simulink model "overhead_crane_control"  (R2022a)
settings: Solver=ode45  StartTime=0.0  StopTime=50  FixedStep=0.001  MaxStep=0.1  MinStep=0.01  RelTol=1e-3  AbsTol=0.01  EnableMultiTasking=on
undefined symbols (not defined in the file): g, k, Kde, Ke, Ku, l, ml, mt, sigbuilder_block
libraries: fuzblock x1
settings Model: Creator=Сергей  LastModifiedBy=clever0ne
settings SolverCC: InitialStep=0.01  ZeroCrossAlgorithm=Adaptive  AlgebraicLoopSolver=TrustRegion
settings DataIOCC: SaveFormat=Array  ReturnWorkspaceOutputs=off
settings OptimizationCC: LifeSpan=inf
settings DebuggingCC: IgnoredZcDiagnostic=none  UnconnectedInputMsg=warning  UnconnectedOutputMsg=warning  UnconnectedLineMsg=warning  AllowSymbolicDim=off  SFUnexpectedBacktrackingDiag=warning  SFNoUnconditionalDefaultTransitionDiag=warning  SFExecutionAtInitializationDiag=none  SFMachineParentedDataDiag=warning  ArithmeticOperatorsInVariantConditions=warning
settings ModelReferenceCC: PropagateSignalLabelsOutOfModel=off
settings SFSimCC: SimUseLocalCustomCode=off  CustomCodeUndefinedFunction=UseInterfaceOnly
settings RTWCC: RTWUseLocalCustomCode=off
settings CodeAppCC: StateflowObjectComments=on
settings GRTTargetCC: TargetLangStandard=C89/C90 (ANSI)
settings ConfigComp: CovMetricSettings=dw  CovSaveCumulativeToWorkspaceVar=on  CovSaveSingleToWorkspaceVar=on  CovExternalEMLEnable=off

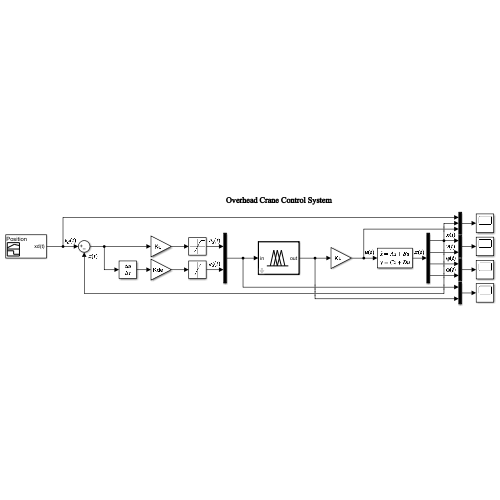
[thumbnail: Simulink's stored preview of the top-level diagram]
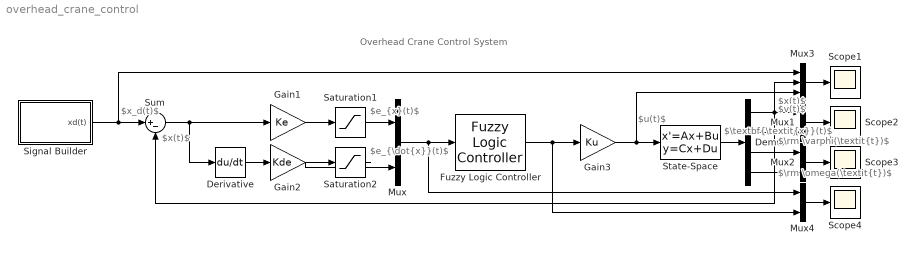
== system overhead_crane_control ==
  note: $\textbf{\textit{x}}(t)$
  note: Overhead Crane Control System
  note: $u(t)$
  note: $x(t)$
  note: $\rm \varphi(\textit{t})$
  note: $v(t)$
  note: $\rm \omega(\textit{t})$
  note: $e_{\dot{x}}(t)$
  note: $e_{x}(t)$
  note: $x(t)$
  note: $x_d(t)$
  Demux : Demux
  Derivative : Derivative
  Fuzzy Logic Controller : fuzblock/Fuzzy Logic  Controller  FIS=fis  OutputSampleNumber=101  DataType=double  FuzzifiedInputs=off  RuleFiringStrengths=off  RuleOutputs=off  AggregatedOutputs=off  SimulateUsing=Interpreted execution  OutOfRangeInputValueMessage=none  NoRuleFiredMessage=none  EmptyOutputFuzzySetMessage=none
  Gain1 : Gain  Gain=Ke
  Gain2 : Gain  Gain=Kde
  Gain3 : Gain  Gain=Ku
  Mux{,1..2,4} (4 alike) : Mux  Inputs=2
  Mux3 : Mux  Inputs=3
  Saturation1 : Saturate  UpperLimit=1  LowerLimit=-1
  Saturation2 : Saturate  UpperLimit=1  LowerLimit=-1
  Scope{1..4} (4 alike) : Scope
  Signal Builder : Subsystem  Tag=STV Subsys  LoadFcn=sigbuilder_block('load');  StartFcn=sigbuilder_block('start');  StopFcn=sigbuilder_block('stop');  ClipboardFcn=sigbuilder_block('clipboard');  mask(Sigbuilder block){tuvar=[0:10]}
      mask help: Simulink:masks:SigbuilderBlock_MD
      mask init:
      | if ~strcmp(get_param(bdroot(gcbh),'SimulationStatus'),'stopped') tuvar = sigbuilder_block('maskInit'); end
      settings: CopyFcn=sigbuilder_block('copy');  DeleteFcn=sigbuilder_block('delete');  ModelCloseFcn=sigbuilder_block('modelClose');  PreSaveFcn=sigbuilder_block('preSave');  PauseFcn=sigbuilder_block('pause');  ContinueFcn=sigbuilder_block('continue');  NameChangeFcn=sigbuilder_block('namechange');  OpenFcn=sigbuilder_block('open',[1347 352.5 550.5 399.75 ]);  CloseFcn=sigbuilder_block('close');
      mask Display: plot(0, 0, 100, 100,[2, 2, 32, 32, 2], [68, 8, 8, 68, 68],[32, 2], [38, 38], [32, 19, 2],[53, 60, 44], [32, 17, 17, 2],[16, 16, 31, 31]);txt = getActiveGroup(gcbh);text(2, 100, txt,'verticalAlignment', 'top');
  State-Space : StateSpace  A=[0, 1, 0, 0; 0, 0, ml*g/mt, 0; 0, 0, 0, 1; 0, 0, -(mt+ml)*g/(mt*l), 0]  B=[0; k/mt; 0; -k/(mt*l)]  C=eye(4)  D=zeros(4, 1)  InitialCondition=0
  Sum : Sum  Inputs=|+-
  wires:
  State-Space/1 -> Demux/1
  Mux1/1 -> Scope2/1
  Mux2/1 -> Scope3/1
  Demux/1 -> Mux1/1, Sum/2, Mux3/2
  Demux/2 -> Mux1/2
  Demux/3 -> Mux2/1
  Demux/4 -> Mux2/2
  Fuzzy Logic Controller/1 -> Gain3/1, Mux4/2
  Gain3/1 -> State-Space/1, Mux3/3
  Mux/1 -> Fuzzy Logic Controller/1, Mux4/1
  Gain2/1 -> Saturation2/1
  Derivative/1 -> Gain2/1
  Sum/1 -> Gain1/1, Derivative/1
  Mux3/1 -> Scope1/1
  Signal Builder/1(xd(t)) -> Mux3/1, Sum/1
  Mux4/1 -> Scope4/1
  Saturation1/1 -> Mux/1
  Gain1/1 -> Saturation1/1
  Saturation2/1 -> Mux/2

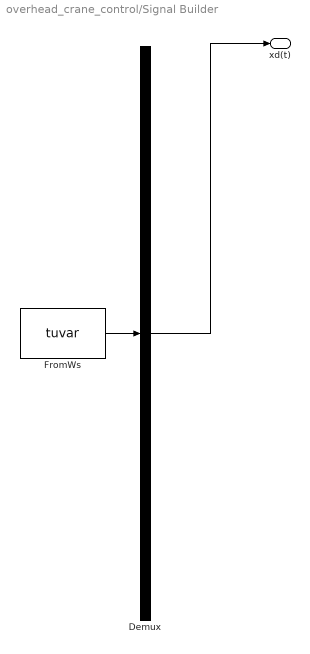
== system overhead_crane_control/Signal Builder ==
  Demux : Demux  Tag=STV Demux  Outputs=1
      settings: DisplayOption=none
  FromWs : FromWorkspace  Tag=STV FromWs  VariableName=tuvar
      SigBuilderData=|
      | common.afterFinalStr = 'Extrapolate'
      | common.sampleTime = 0
      | dataSet.timeRange = [0 300]
      | dataSet.name = 'Position'
      | sbobj.Groups.Name = 'Position'
      | sbobj.Groups.Signals.Name = 'xd(t)'
      | sbobj.Groups.Signals.XData = [0 10 10 100 100 200 200 300]
      | sbobj.Groups.Signals.YData = [0 0 40 40 20 20 0 0]
      | sbobj.Groups.TimeRange = [0 300]
  xd(t) : Outport  Tag=STV Outport
  wires:
  Demux/1 -> xd(t)/1
  FromWs/1 -> Demux/1
